simulink model "LQR_Model"  (R2015b)
settings: Solver=VariableStepAuto  StartTime=0.0  StopTime=100  RelTol=1e-3
values from neighbouring files (symbols this model uses):
  H = (sys_d.a * P * sys_d.c' + R_12) * inv(sys_d.c * P * sys_d.c' + R_2)    [Kalman.m]    (also in matlab.mat = [-0.750018076363 0.0551905208319 0.6347810371])
  K = [0.0479753648602 0.034211028751 0.00928748155312]    [matlab.mat]
  LQR = [-0.566321569976 0.00826847649943 0 9.99988971029 9.8593256098 -0.500173757981 0 79.9164329174 -0.0826847649943 9.99988971029 0 174.999862655 ... (16 elements, 4x4)]    [matlab.mat]
undefined symbols (not defined in the file or in its folder): sys_d
settings Model: Creator=Jcama  LastModifiedBy=Jcama

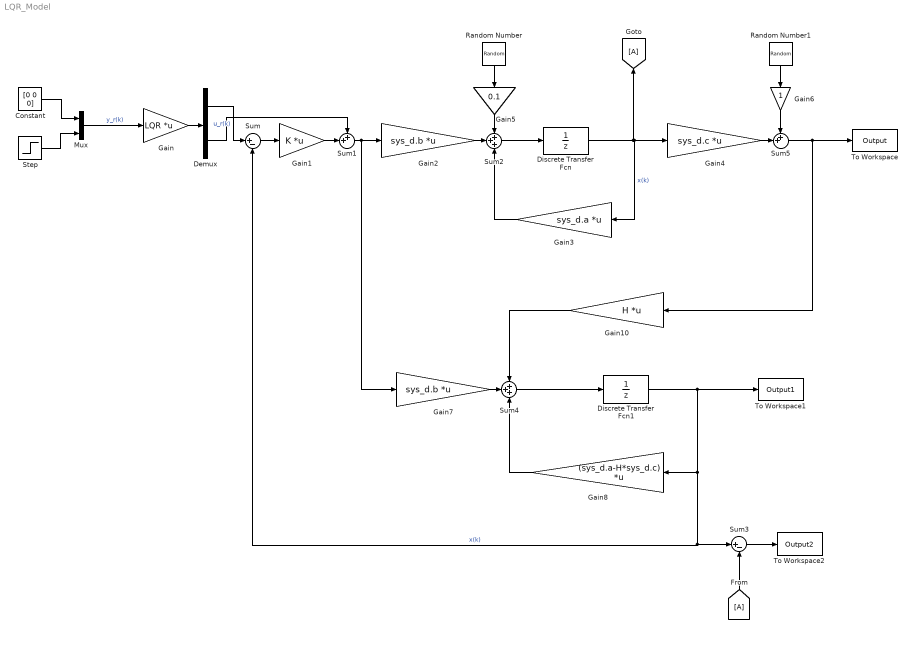
== system LQR_Model ==
  Constant : Constant  Value=[0 0 0]
  Demux : Demux  Outputs=[3 1]
  Discrete Transfer Fcn : DiscreteTransferFcn  Denominator=[1 0]
  Discrete Transfer Fcn1 : DiscreteTransferFcn  Denominator=[1 0]
  Gain : Gain  Gain=LQR  Multiplication=Matrix(K*u)
  Gain1 : Gain  Gain=K  Multiplication=Matrix(K*u)
  Gain10 : Gain  Gain=H  Multiplication=Matrix(K*u)
  Gain2 : Gain  Gain=sys_d.b  Multiplication=Matrix(K*u)
  Gain3 : Gain  Gain=sys_d.a  Multiplication=Matrix(K*u)
  Gain4 : Gain  Gain=sys_d.c  Multiplication=Matrix(K*u)
  Gain5 : Gain  Gain=0.1
  Gain6 : Gain
  Gain7 : Gain  Gain=sys_d.b  Multiplication=Matrix(K*u)
  Gain8 : Gain  Gain=(sys_d.a-H*sys_d.c)  Multiplication=Matrix(K*u)
  Mux : Mux  Inputs=2
  Random Number : RandomNumber  Variance=0.6  SampleTime=0.1
  Random Number1 : RandomNumber  Variance=0.6  SampleTime=0.1
  Step : Step  After=80  SampleTime=0.1
  Sum : Sum  Inputs=|+-
  Sum1 : Sum  Inputs=++|
  Sum2 : Sum  Inputs=+++
  Sum3 : Sum  Inputs=|+-
  Sum4 : Sum  Inputs=+++
  Sum5 : Sum  Inputs=++|
  To Workspace : ToWorkspace  VariableName=Output  SaveFormat=Timeseries  SampleTime=0.1
  To Workspace1 : ToWorkspace  VariableName=Output1  SaveFormat=Timeseries  SampleTime=0.1
  To Workspace2 : ToWorkspace  VariableName=Output2  SaveFormat=Timeseries  SampleTime=0.1
  wires:
  Gain/1 -> Demux/1
  Sum/1 -> Gain1/1
  Gain1/1 -> Sum1/2
  Sum2/1 -> Discrete Transfer Fcn/1
  Discrete Transfer Fcn/1 -> Gain4/1, Gain3/1, [A]  "x(k)"
  Gain2/1 -> Sum2/2
  Gain3/1 -> Sum2/3
  Gain5/1 -> Sum2/1
  Random Number/1 -> Gain5/1
  Mux/1 -> Gain/1  "y_r(k)"
  Demux/2 -> Sum1/1
  Demux/1 -> Sum/1  "u_r(k)"
  Constant/1 -> Mux/1
  Step/1 -> Mux/2
  Sum1/1 -> Gain2/1, Gain7/1
  Sum4/1 -> Discrete Transfer Fcn1/1
  Gain7/1 -> Sum4/2
  Gain8/1 -> Sum4/3
  Gain10/1 -> Sum4/1
  Discrete Transfer Fcn1/1 -> Gain8/1, Sum/2, Sum3/1, To Workspace1/1  "x(k)"
  Sum3/1 -> To Workspace2/1
  [A] -> Sum3/2
  Gain4/1 -> Sum5/2
  Sum5/1 -> Gain10/1, To Workspace/1
  Gain6/1 -> Sum5/1
  Random Number1/1 -> Gain6/1
